simulink model "task_4_scheme"  (R2024a)
settings: Solver=FixedStepAuto  StartTime=0.0  StopTime=20.0  FixedStep=0.001  RelTol=1e-3
settings Model: Creator=alexe  LastModifiedBy=alexe

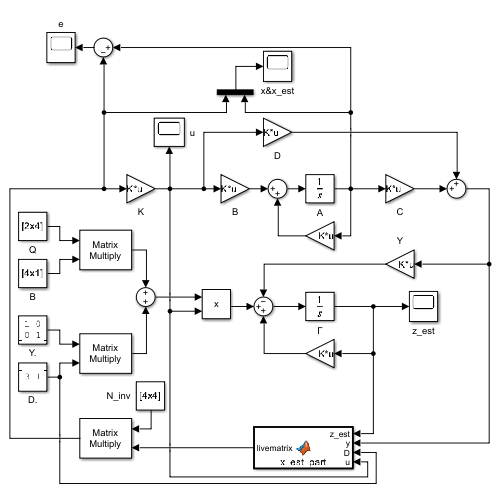
[thumbnail: Simulink's stored preview of the top-level diagram]
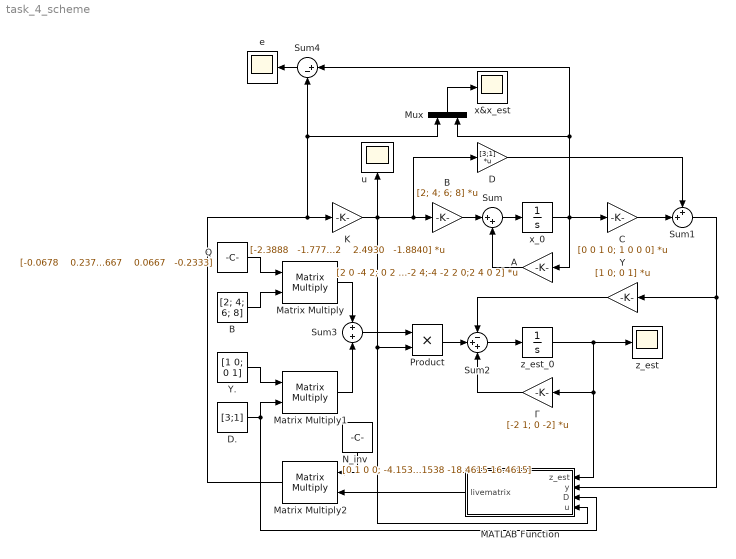
== system task_4_scheme ==
  A : Gain  Gain=[2 0 -4 2; 0 2 -2 4;-4 -2 2 0;2 4 0 2]  Multiplication=Matrix(K*u)
  B : Gain  Gain=[2; 4; 6; 8]  Multiplication=Matrix(K*u)
  C : Gain  Gain=[0 0 1 0; 1 0 0 0]  Multiplication=Matrix(K*u)
  D : Gain  Gain=[3;1]  Multiplication=Matrix(K*u)
  D. : Constant  Value=[3;1]
  K : Gain  Gain="[-2.3888   -1.7772    2.4930   -1.8840]"  Multiplication=Matrix(K*u)
  MATLAB Function : MATLAB Function  TreatAsAtomicUnit=on
  Matrix Multiply : Product  Multiplication=Matrix(*)
  Matrix Multiply1 : Product  Multiplication=Matrix(*)
  Matrix Multiply2 : Product  Multiplication=Matrix(*)
  Mux : Mux  Inputs=2
  N_inv : Constant  Value="[0 1 0 0; -4.1538 0.1154  -16.1538 18.1538; 1 0 0 0; -4.4615 -0.1538 -18.4615 16.4615]"
  Product : Product
  Q : Constant  Value="[-0.0678    0.2378   -0.1822   -0.2622; -0.0667    0.2667    0.0667   -0.2333]"
  Sum : Sum  Inputs=|++
  Sum1 : Sum  Inputs=++|
  Sum2 : Sum  Inputs=-++
  Sum3 : Sum  Inputs=+|+
  Sum4 : Sum  Inputs=|+-
  Y : Gain  Gain=[1 0; 0 1]  Multiplication=Matrix(K*u)
  Y. : Constant  Value=[1 0; 0 1]
  e : Scope
  u : Scope
  x&x_est : Scope
  x_0 : Integrator  InitialCondition=[1;1;1;1]
  z_est : Scope
  z_est_0 : Integrator  InitialCondition=[0; 0]
  В : Constant  Value=[2; 4; 6; 8]
  Г : Gain  Gain=[-2 1; 0 -2]  Multiplication=Matrix(K*u)
  wires:
  x_0/1 -> Sum4/1, Mux/2, C/1, A/1
  B/1 -> Sum/1
  Sum/1 -> x_0/1
  A/1 -> Sum/2
  K/1 -> D/1, B/1, u/1, MATLAB Function/4(u), Product/2
  C/1 -> Sum1/2
  D/1 -> Sum1/1
  Q/1 -> Matrix Multiply/1
  В/1 -> Matrix Multiply/2
  Y./1 -> Matrix Multiply1/1
  D./1 -> MATLAB Function/3(D), Matrix Multiply1/2
  Sum2/1 -> z_est_0/1
  Matrix Multiply/1 -> Sum3/1
  Matrix Multiply1/1 -> Sum3/2
  Sum3/1 -> Product/1
  Product/1 -> Sum2/2
  Г/1 -> Sum2/3
  Y/1 -> Sum2/1
  Matrix Multiply2/1 -> K/1, Mux/1, Sum4/2
  z_est_0/1 -> Г/1, MATLAB Function/1(z_est), z_est/1
  Mux/1 -> x&x_est/1
  Sum4/1 -> e/1
  N_inv/1 -> Matrix Multiply2/1
  MATLAB Function/1(livematrix) -> Matrix Multiply2/2
  Sum1/1 -> MATLAB Function/2(y), Y/1

== matlab function task_4_scheme/MATLAB Function ==
  data: z_est input; y input; D input; u input; livematrix output
function livematrix = x_est_part(z_est, y, D, u)
livematrix = [y - D * u; z_est];
end
